simulink model "LPV_pump_pipe"  (R2019b)
settings: Solver=VariableStepAuto  StartTime=0.0  StopTime=t(end)  RelTol=1e-3
undefined symbols (not defined in the file or in its folder): magnitude, th1, th2, Ts, UseEstimatedP
libraries: cstblocks x1
settings Model: Creator=The MathWorks, Inc.  LastModifiedBy=The MathWorks, Inc.
settings DataIOCC: SaveOutput=off  DSMLogging=off  SaveTime=off  ReturnWorkspaceOutputs=off
settings DebuggingCC: ArithmeticOperatorsInVariantConditions=warning
settings SFSimCC: SimUseLocalCustomCode=off  CustomCodeUndefinedFunction=UseInterfaceOnly
settings RTWCC: RTWUseLocalCustomCode=off

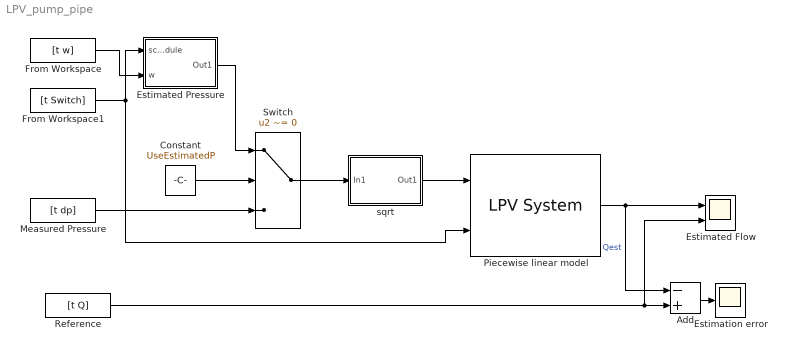
== system LPV_pump_pipe ==
  Add : Sum  Inputs=-+
  Constant : Constant  Value=UseEstimatedP
  Estimated Pressure : Subsystem
  Estimated Flow : Scope  NumInputPorts=2
  Estimation error : Scope
  From Workspace : FromWorkspace  VariableName=[t w]  SampleTime=Ts  OutputAfterFinalValue=Holding final value
  From Workspace1 : FromWorkspace  VariableName=[t Switch]  SampleTime=Ts  Interpolate=off  OutputAfterFinalValue=Holding final value
  Measured Pressure : FromWorkspace  VariableName=[t dp]  SampleTime=Ts
  Piecewise linear model : cstblocks/Linear Parameter Varying/LPV System  sys=sys  x0=0  uOffset=0  yOffset=offset  xOffset=offset  opEquilOption=on  dxOffset=0  sysFixedOption=Use the first model in state-space array  sysFixed=[]  AFixed=false  BFixed=false  CFixed=false  DFixed=false  uDelayFixed=false  yDelayFixed=false  iDelayFixed=false  IMethod=Nearest  EMethod=Clip  IndexSearch=Binary search  IndexBegin=on  OutputX=off  OutputXdot=off  OutputLTI=off  OutputOP=off  DataType=double  SimMode=Interpreted execution  InitBufferSize=1024  FixedBuffer=off
      settings: SourceProductName=Control System Toolbox  SourceProductBaseCode=CT
  Reference : FromWorkspace  VariableName=[t Q]  SampleTime=Ts  OutputAfterFinalValue=Holding final value
  Switch : Switch  Criteria=u2 ~= 0
  sqrt : Subsystem
  wires:
  From Workspace1/1 -> Piecewise linear model/2, Estimated Pressure/1(schedule)
  From Workspace/1 -> Estimated Pressure/2(w)
  sqrt/1(Out1) -> Piecewise linear model/1
  Estimated Pressure/1(Out1) -> Switch/1
  Measured Pressure/1 -> Switch/3
  Switch/1 -> sqrt/1(In1)
  Piecewise linear model/1 -> Add/1, Estimated Flow/1  "Qest"
  Reference/1 -> Estimated Flow/2, Add/2
  Add/1 -> Estimation error/1
  Constant/1 -> Switch/2

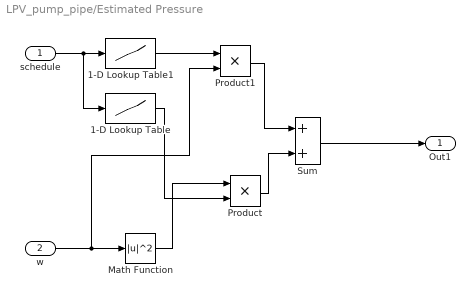
== system LPV_pump_pipe/Estimated Pressure ==
  schedule : Inport
  w : Inport  Port=2
  1-D Lookup Table : Lookup_n-D  NumberOfTableDimensions=1  BreakpointsForDimension1=[1 2 3]  Table=th1  InternalRulePriority=Speed  RndMeth=Simplest  InputSameDT=on
  1-D Lookup Table1 : Lookup_n-D  NumberOfTableDimensions=1  BreakpointsForDimension1=[1 2 3]  Table=th2  InternalRulePriority=Speed  RndMeth=Simplest  InputSameDT=on
  Math Function : Math  Operator=magnitude^2  SaturateOnIntegerOverflow=on
  Product : Product
  Product1 : Product
  Sum : Sum
  Out1 : Outport  VectorParamsAs1DForOutWhenUnconnected=off
  wires:
  w/1 -> Product1/2, Math Function/1
  1-D Lookup Table1/1 -> Product1/1
  1-D Lookup Table/1 -> Product/2
  Product/1 -> Sum/2
  schedule/1 -> 1-D Lookup Table/1, 1-D Lookup Table1/1
  Math Function/1 -> Product/1
  Product1/1 -> Sum/1
  Sum/1 -> Out1/1

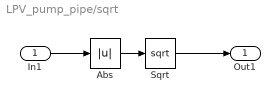
== system LPV_pump_pipe/sqrt ==
  In1 : Inport
  Abs : Abs
  Sqrt : Sqrt  SaturateOnIntegerOverflow=on
  Out1 : Outport  VectorParamsAs1DForOutWhenUnconnected=off
  wires:
  Abs/1 -> Sqrt/1
  In1/1 -> Abs/1
  Sqrt/1 -> Out1/1
